simulink model "2025.1.21.methods"  (R2023a)
settings: Solver=ode4  StartTime=0.0  StopTime=40  FixedStep=dt  RelTol=1e-3
values from neighbouring files (symbols this model uses):
  AgN = Ag    [Copy_of_New_Ns.m]    (also in 旧数值子结构.m = zeros(ndof,1))
  C_phys_5dof = C    [旧静力凝聚.m]
  CNrt = CRrt    [Copy_of_New_Ns.m]    (also in 旧数值子结构.m)
  FN = zeros(15,1)    [Copy_of_New_Ns.m]    (also in 旧数值子结构.m = zeros(ndof,1))
  K_phys_5dof = K    [旧静力凝聚.m]
  KNbar_inv = inv(KNbar)    [Copy_of_New_Ns.m]    (also in 旧数值子结构.m)
  Koo = K(3:end,3:end)    [旧静力凝聚.m]
  Kot = K(3:end,1:2)    [旧静力凝聚.m]
  lN = l    [Copy_of_New_Ns.m]    (also in 旧数值子结构.m = zeros(ndof,1))
  M_phys_5dof = M    [旧静力凝聚.m]
  MNrt = diag([M1 1e-5 M6 M3 M2 M4 1e-5 M6 M3 M2 M1 M2 M3 M3 M2])    [Copy_of_New_Ns.m]    (also in 旧数值子结构.m = csvread("FE_Model/REF_SAP2000_Model/M_matrix.csv"))
  RNbar = zeros(15,1)    [Copy_of_New_Ns.m]    (also in 旧数值子结构.m = zeros(ndof,1))
undefined symbols (not defined in the file or in its folder): a0, a1, a2, a3, a4, a5, a6, a7, A_cplant, alpha1, alpha2, B_cplant, C_cplant, D_cplant, Dd_ss, delay, Ds_ss, dt, dv1, dv2, EQ_intensity, EQ_sw, Gnd_ss, Gns_ss, Hs1, Hs2, k3, k4, k6, K_lqr, KE, Mren, Muu, Phi_u2, Seed_snr
libraries: simulink x2, slpidlib x2, sldrtlib x1
(part 2 of 2)

== matlab function 2025.1.21.methods/1阶1/ 数值子结构2/MATLAB Function1 ==
  data: U27_MA output; V27_MA output; A27_MA output; Theta21_MA output; VTheta21_MA output; ATheta21_MA output; Theta29_MA output; VTheta29_MA output; ATheta29_MA output; U2nd output; Theta2nd output; U3rd output; Theta3rd output; U1 output; Vel1 output; Acc1 output; accel_grd input; FB_force27 input; FB_moment29 input; FB_moment21 input; Kbar_inv input; MNrt input; CNrt input; Ag input; l input; Rbar input; F input; U0 input; Vel0 input; Acc0 input; a0 parameter; a1 parameter; a2 parameter; a3 parameter; a4 parameter; a5 parameter; a6 parameter; a7 parameter; Rbar output
function [U27_MA,V27_MA,A27_MA,Theta21_MA,VTheta21_MA,ATheta21_MA,Theta29_MA,VTheta29_MA,ATheta29_MA,U2nd,Theta2nd,U3rd,Theta3rd,U1,Vel1,Acc1,Rbar]=...
    fcn(accel_grd,FB_force27,FB_moment29,FB_moment21,Kbar_inv, MNrt, CNrt,Ag,l,Rbar,F,...
    U0,Vel0,Acc0, a0, a1, a2, a3, a4, a5, a6, a7)
             
             
    % ============================
	% *  Update next iteration   *
	% ============================
    ndof = length(Kbar_inv);
    U1   = zeros(ndof,1);
    Vel1 = zeros(ndof,1);
    Acc1 = zeros(ndof,1);
    
    U27_MA = 0;
    V27_MA = 0;
    A27_MA = 0;

    Theta21_MA = 0;
    VTheta21_MA = 0;
    ATheta21_MA = 0;
% 
%     U6_MA = 0;
%     V6_MA = 0;
%     A6_MA = 0;
    U2nd = 0 ;              %Displacement 2nd story, node 12, DOF 26
    Theta2nd = 0;          %Rotation 2nd story, node 12, DOF 22
    U3rd = 0;              %Displacement 3rd story, node 16, DOF 13
    Theta3rd = 0;           %Rotation 3rd story, node 16, DOF 3


    Theta29_MA = 0;
    VTheta29_MA = 0;
    ATheta29_MA = 0;

    % ============================
	% *  Feedback Force / Moment *
	% ============================
    F(27) = FB_force27;
    F(21) = FB_moment21;
    F(29) = FB_moment29;

    % ==========================
	% *     Update Matrices    *
	% ==========================
    Ag(:)  = accel_grd * l;
    
   	% ==========================
	% * 	  Form Rbar  	   *
	% ==========================
	Rbar = ( (MNrt * ((a0*U0)+(a2*Vel0)+(a3*Acc0))) + ...
		     (CNrt * ((a1*U0)+(a4*Vel0)+(a5*Acc0))) - F - (MNrt * Ag) );
    
    % ==========================
	% * Solve for Displacement *
	% ==========================
	U1 = Kbar_inv * Rbar;
    
	% ============================
	% * Compute Velocity & Accel *
	% ============================
	Acc1=a0*(U1-U0)-a2*Vel0-a3*Acc0;
	Vel1=Vel0+a7*Acc1+a6*Acc0; 

	% ============================
	% *    Output u1 and theta   *
	% ============================
    U27_MA    = U1(27);
    V27_MA    = Vel1(27);
    A27_MA    = Acc1(27);    

%     U6_MA    = U1(27);
%     V6_MA    = Vel1(27);
%     A6_MA    = Acc1(27);

    Theta21_MA = U1(21);
    VTheta21_MA = Vel1(21);
    ATheta21_MA = Acc1(21);

    Theta29_MA = U1(29);
    VTheta29_MA = Vel1(29);
    ATheta29_MA = Acc1(29);
    
    % ADDED by Johnny
    U2nd = U1(26);              %Displacement 2nd story, node 12, DOF 26
    Theta2nd = U1(22);          %Rotation 2nd story, node 12, DOF 22
    U3rd = U1(13);              %Displacement 3rd story, node 16, DOF 13
    Theta3rd = U1(3);           %Rotation 3rd story, node 16, DOF 3

end
